simulink model "Cowley_315Exam2TakeHomeSim3"  (R2020b)
settings: Solver=FixedStepAuto  StartTime=0.0  StopTime=20  FixedStep=0.01  RelTol=1e-3
libraries: simulink x2
settings Model: Creator=mattcowley  LastModifiedBy=mattcowley

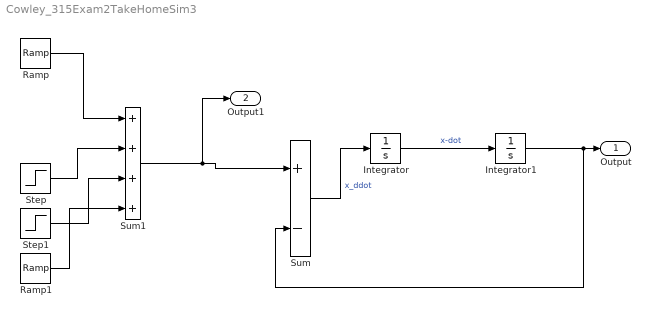
== system Cowley_315Exam2TakeHomeSim3 ==
  Integrator : Integrator
  Integrator1 : Integrator
  Ramp : simulink/Sources/Ramp  slope=1  start=0  InitialOutput=0
  Ramp1 : simulink/Sources/Ramp  slope=-1  start=pi  InitialOutput=0
  Step : Step  Time=pi  After=1-pi  SampleTime=0
  Step1 : Step  Time=2*pi  After=-1  SampleTime=0
  Sum : Sum  Inputs=+-
  Sum1 : Sum  Inputs=++++
  Output : Outport  SignalName=x
  Output1 : Outport  Port=2  SignalName=F
  wires:
  Integrator/1 -> Integrator1/1  "x-dot"
  Integrator1/1 -> Sum/2, Output/1
  Sum/1 -> Integrator/1  "x_ddot"
  Sum1/1 -> Output1/1, Sum/1
  Ramp/1 -> Sum1/1
  Step/1 -> Sum1/2
  Step1/1 -> Sum1/3
  Ramp1/1 -> Sum1/4
